simulink model "detect_test"  (R2023a)
settings: Solver=VariableStepAuto  StartTime=0.0  StopTime=.0025  RelTol=1e-3
PostLoadFcn:
  | detect_test_init
undefined symbols (not defined in the file): detect_SingleWindow, S, SingleWindow, SR, vsva2197, xcvc1902
libraries: dspsrcs4 x2, hdlsllib x1, dspxfrm3 x1, vmcUtilities x1, aieBasic x1
settings Model: Creator=ss112260  LastModifiedBy=robg
settings ModelReferenceCC: EnableRefExpFcnMdlSchedulingChecks=on

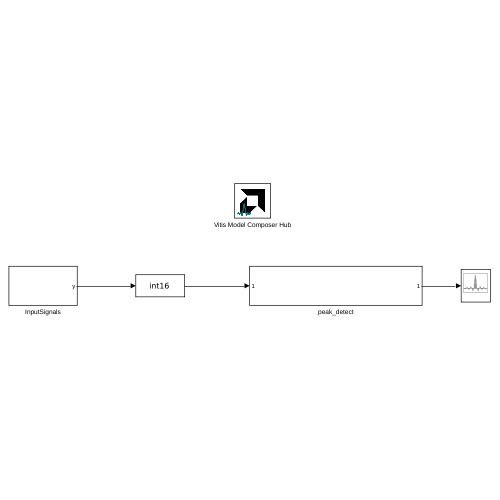
[thumbnail: Simulink's stored preview of the top-level diagram]
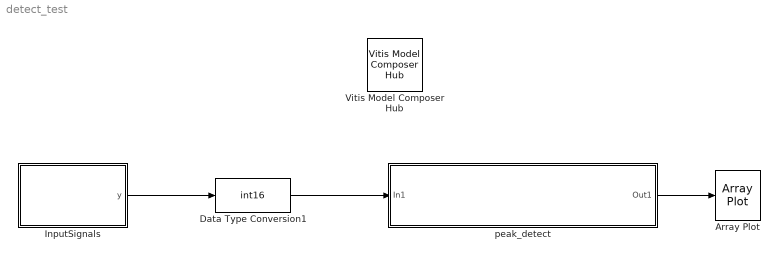
== system detect_test ==
  Array Plot : ArrayPlot  WindowPosition=[1625.000000,180.000000,891.000000,563.000000,]  Visible=on  YLimits=[-37.375,336.375]
  Data Type Conversion1 : DataTypeConversion  OutDataTypeStr=int16  SaturateOnIntegerOverflow=off  RndMeth=Floor
  InputSignals : Subsystem
  Vitis Model Composer Hub : vmcUtilities/Vitis Model Composer Hub  Tag=genX  CodeGeneration=off  SubsystemName=avg_power  StartColumn=1  NumberOfColumns=1  TargetDirectory=./code_1  exportDesign=off  analyzeDesign=off  validateDesignOnHw=off  ExportType=AI Engines  IpVendor=xilinx.com  IpLibrary=hls  IpVersion=1.0  IpHWLanguage=Verilog  AieCompilerOptions={}  AieSimulatorOptions={}  CreateTestbench=on  TestbenchStackSize=10  RunRtlSim=off  RunCSim=off  RunAieSim=on  AieSimTimeout=50000  RunAieSimProfiling=on  LaunchVitisAnalyzer=on  PlotOutput=on  RunX86Sim=off  X86SimTimeout=10  GenHwImage=off  GenLibadfXo=off  GenHwValidationCode=off  PlatformType=Specify Platform  Platform=/home/ss112260/Programs/tools/Xilinx/Vitis/2022.2/base_platforms/xilinx_vck190_base_202220_1/xilinx_vck190_base_202220_1.xpfm  HwSystemType=Baremetal  HwValidationTarget=hw  ProjDevice=Versal VCK190 Evaluation Platform (xcvc1902-vsva2197-2MP-e-S)  ProjDevicePart=xcvc1902-vsva2197-2MP-e-S  AIEType=AIE  SamplePeriod=-1  ClockFrequency=200  DataPathParallelism=1  xilinxfamily=versalaicore  part=xcvc1902  speed=-2MP-e-S  package=vsva2197  directory=./netlist  testbench=off  incr_netlist=off  synthesis_tool=Vivado  clock_wrapper=Clock Enables  dbl_ovrd=According to Block Masks  dcm_input_clock_period=10  sysclk_period=10  simulink_period=1  eval_field=0  LogFileName=''  NThreads=4
  peak_detect : Subsystem
  wires:
  Data Type Conversion1/1 -> peak_detect/1(In1)
  peak_detect/1(Out1) -> Array Plot/1
  InputSignals/1(y) -> Data Type Conversion1/1

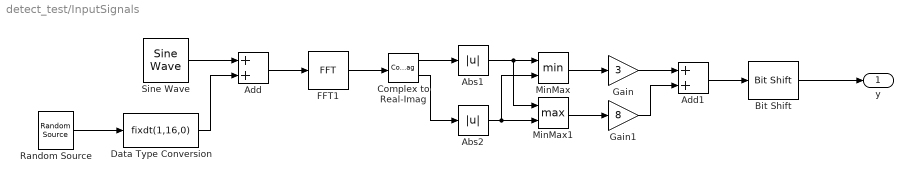
== system detect_test/InputSignals ==
  Abs1 : Abs  SaturateOnIntegerOverflow=off
  Abs2 : Abs  SaturateOnIntegerOverflow=off
  Add : Sum
  Add1 : Sum  AccumDataTypeStr=fixdt(1,16,0)
  Bit Shift : hdlsllib/Logic and Bit Operations/Bit Shift  mode=Shift Right Logical  N=3
  Complex to Real-Imag : ComplexToRealImag
  Data Type Conversion : DataTypeConversion  OutDataTypeStr=fixdt(1,16,0)  SaturateOnIntegerOverflow=off  RndMeth=Floor
  FFT1 : dspxfrm3/FFT  FFTImplementation=Auto  CompMethod=Table lookup  TableOpt=NEW  TableOptActive=Speed  BitRevOrder=off  Normalize=on  InheritFFTLength=off  FFTLength=frameSize  WrapInput=off  roundingMode=Floor  overflowMode=on  firstCoeffDataTypeStr=Inherit: Same word length as input  firstCoeffLastDataTypeStr=Inherit: Same word length as input  outputMode=Binary point scaling  outputWordLength=16  outputFracLength=0  outputDataTypeStr=fixdt(1,16,0)  outputMin=[]  outputMax=[]  outputLastDataTypeStr=fixdt(1,16,0)
  Gain : Gain  Gain=3  ParamDataTypeStr=fixdt(1,16,0)
  Gain1 : Gain  Gain=8  OutDataTypeStr=int16
  MinMax : MinMax  Inputs=2
  MinMax1 : MinMax  Function=max  Inputs=2
  Random Source : dspsrcs4/Random Source  SrcType=Uniform  NormMethod=Ziggurat  CltLength=12  MinVal=-16  MaxVal=16  MeanVal=0  VarVal=1  RepMode=Not repeatable  rawSeed=1  IsInherit=off  SampMode=Discrete  SampTime=1/SR  SampFrame=frameSize  DataType=Double  OutComplex=Complex  OutputFrames=off
  Sine Wave : dspsrcs4/Sine Wave  Amplitude=512  Frequency=25e6  Phase=0  SampleMode=Discrete  OutComplex=Complex  CompMethod=Table lookup  TableSize=Speed  SampleTime=1/SR  SamplesPerFrame=frameSize  ResetState=Restart at time zero  OutputFrames=off  dataType=Fixed-point  wordLen=16  udDataType=sfix(16)  fracBitsMode=User-defined  numFracBits=0  OutDataTypeStr=fixdt(1,16,0)  LastOutDataTypeStr=fixdt(1,16,0)
  y : Outport
  wires:
  Data Type Conversion/1 -> Add/2
  Gain1/1 -> Add1/2
  Add/1 -> FFT1/1
  MinMax1/1 -> Gain1/1
  Sine Wave/1 -> Add/1
  Complex to Real-Imag/1 -> Abs1/1
  Abs2/1 -> MinMax/2, MinMax1/2
  Add1/1 -> Bit Shift/1
  Gain/1 -> Add1/1
  Bit Shift/1 -> y/1
  FFT1/1 -> Complex to Real-Imag/1
  Random Source/1 -> Data Type Conversion/1
  Complex to Real-Imag/2 -> Abs2/1
  MinMax/1 -> Gain/1
  Abs1/1 -> MinMax1/1, MinMax/1

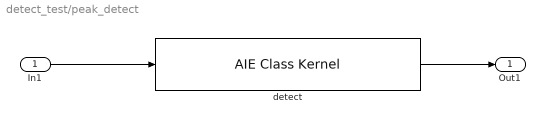
== system detect_test/peak_detect ==
  In1 : Inport
  detect : aieBasic/AIE Class Kernel  KernelAllAttrs=|  PortNames={'iwinPower'; 'owinDetect'}  PortSerializedTypes={'{Q2{P{Tinput_window{1{t{Bi16}}}}}}'; '{Q2{P{Toutput_window{1{t{Bi32}}}}}}'}  PortWindowSizes={2.048000000000000000e+03; 2.048000000000000000e+03}  PortWindowMargins={0.000000000000000000e+00; 0.000000000000000000e+00}  PortSynchronicities={'sync', 'sync'}  PortSignalSizes={0.000000000000000000e+00; 0.000000000000000000e+00}  ClassTemplateSpecKind=implicit  ClassTemplateParamNames={'NUMSAMPLES'; 'AVERAGE'}  ClassTemplateParamKinds={'nontype'; 'nontype'}  ClassTemplateParamTypes={'int'; 'int'}  ClassTemplateParamValues={'2048', '4'}  ClassCtorParamNames={}  ClassCtorParamSerializedTypes={}  ClassCtorParamValues={}  ClassIndex=1  ClassCtorIndex=0  ClassTabVisible=on  ClassTemplateParamsVisible=on  ClassCtorDeclVisible=off  ClassCtorParamsVisible=off  FunctionTabVisible=on  FunctionDecl=|  PortAttrs={ 'input', 'iwinPower', 'input_window_int16 * restrict', 'frameSize', '0', 'sync', ''; 'output', 'owinDetect', 'output_window_int32 * restrict', 'frameSize', '', 'sync', '' }  PortAttrsEnables={'off', 'off', 'off', 'on', 'on', 'on', 'off';'off', 'off', 'off', 'on', 'off', 'on', 'off'}  SampleTime=-1  ClassDeclTypeOptions=|  ClassDecl=|  ClassTemplateParams={ 'NUMSAMPLES', 'int', 'frameSize'; 'AVERAGE', 'int', '4' }  ClassTemplateParamsEnables={'off', 'off', 'on';'off', 'off', 'on'}  ClassCtorDeclTypeOptions=C[1 1]@t7@<empty>  ClassCtorDecl=<empty>  ClassCtorParams={}  KernelHeaderFile=detectSingleWindow.h  KernelClassName=SingleWindow::detect_SingleWindow  KernelFunction=detect  KernelSourceFile=detectSingleWindow.cpp  KernelSearchPaths={}  PreProcOptions={}  blockJsonConstraints=[]
      KernelAllAttrs=|
      | s[12;12;9;9;19;14;21;23;21;23;24;21;15;17;12;24;26;26;26;27;28;9;21;23;23;23;24;25;14;19;19;29]@FunctionNameDeclFileNamePortNamesPortTypesPortSerializedTypesPortDirectionsPortWindowSizeEnablesPortWindowMarginEnablesPortBufferSizeEnablesPortBufferMarginEnablesPortSynchronicityEnablesPortSignalSizeEnablesPortBufferSizesPortBufferMarginsFunctionDeclFunctionTemplateSpecKindFunctionTemplateParamNamesFunctionTemplateParamKindsFunctionTemplateParamTypesFunctionTemplateParamValuesFunctionTemplateParamEnablesClassDeclClassTemplateSpecKindClassTemplateParamNamesClassTemplateParamKindsClassTemplateParamTypesClassTemplateParamValuesClassTemplateParamEnablesClassCtorDeclsClassCtorParamNamesClassCtorParamTypesClassCtorParamSerializedTypes[1 1]@C[32 1]@t6@detectt37@../../aie_kernel/detectSingleWindow.hC[2 1]@t9@iwinPowert10@owinDetectC[2 1]@t29@input_window_int16 * restrictt30@output_window_int32 * restrictC[2 1]@t34@{Q2{P{Tinput_window{1{t{Bi16}}}}}}t35@{Q2{P{Toutput_window{1{t{Bi32}}}}}}C[2 1]@t5@inputt6@outputC[2 1]@l1@l1@C[2 1]@l1@l0@C[2 1]@l0@l0@C[2 1]@l0@l0@C[2 1]@l1@l1@C[2 1]@l0@l0@C[2 1]@nnC[2 1]@nnt187@namespace SingleWindow {
      | template < int NUMSAMPLES, int AVERAGE > 
      | void detect_SingleWindow::
      | detect(input_window_int16 * restrict iwinPower, output_window_int32 * restrict owinDetect);
      | }t4@nonee[0 1]@e[0 1]@e[0 1]@e[0 1]@e[0 1]@t94@namespace SingleWindow {
      | template < int NUMSAMPLES, int AVERAGE > class detect_SingleWindow;
      | }t8@implicitC[2 1]@t10@NUMSAMPLESt7@AVERAGEC[2 1]@t7@nontypet7@nontypeC[2 1]@t3@intt3@intC[2 1]@nnC[2 1]@l1@l1@e[0 1]@e[0 1]@e[0 1]@e[0 1]@
      FunctionDecl=|
      | namespace SingleWindow {
      | template < int NUMSAMPLES, int AVERAGE > 
      | void detect_SingleWindow::
      | detect(input_window_int16 * restrict iwinPower, output_window_int32 * restrict owinDetect);
      | }
      ClassDeclTypeOptions=|
      | C[1 1]@t94@namespace SingleWindow {
      | template < int NUMSAMPLES, int AVERAGE > class detect_SingleWindow;
      | }
      ClassDecl=|
      | namespace SingleWindow {
      | template < int NUMSAMPLES, int AVERAGE > class detect_SingleWindow;
      | }
  Out1 : Outport
  wires:
  In1/1 -> detect/1
  detect/1 -> Out1/1
